simulink model "lugre_stick_slip"  (R2023a)
settings: Solver=FixedStepAuto  StartTime=0.0  StopTime=50  FixedStep=1e-4  RelTol=1e-3
values from neighbouring files (symbols this model uses):
  Ac = [0 1; 0 0]    [LuGre_parameters.m]
  alpha = 1    [LuGre_parameters.m]
  Fc = 2.94    [LuGre_parameters.m]
  Fs = 5.88    [LuGre_parameters.m]
  k = 2    [LuGre_parameters.m]
  Kstfb = [place(Ac,Bc,[-35,-30]),0]    [LuGre_parameters.m]
  m = 1    [LuGre_parameters.m]
  sigma0 = 2900    [LuGre_parameters.m]
  sigma1 = 107    [LuGre_parameters.m]
  sigma2 = 0    [LuGre_parameters.m]
  vs = 0.1    [LuGre_parameters.m]
libraries: slpidlib x1, simulink x1
settings Model: Creator=Alex  LastModifiedBy=Alex

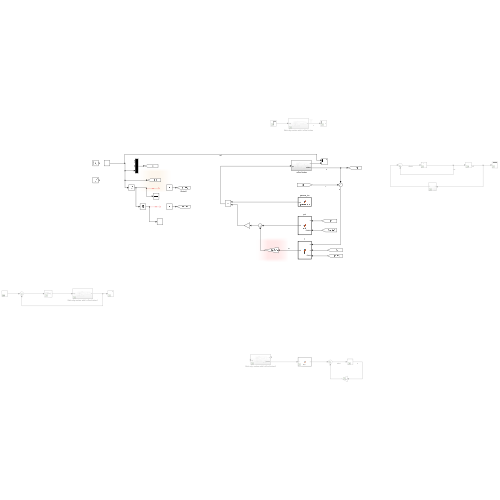
[thumbnail: Simulink's stored preview of the top-level diagram]
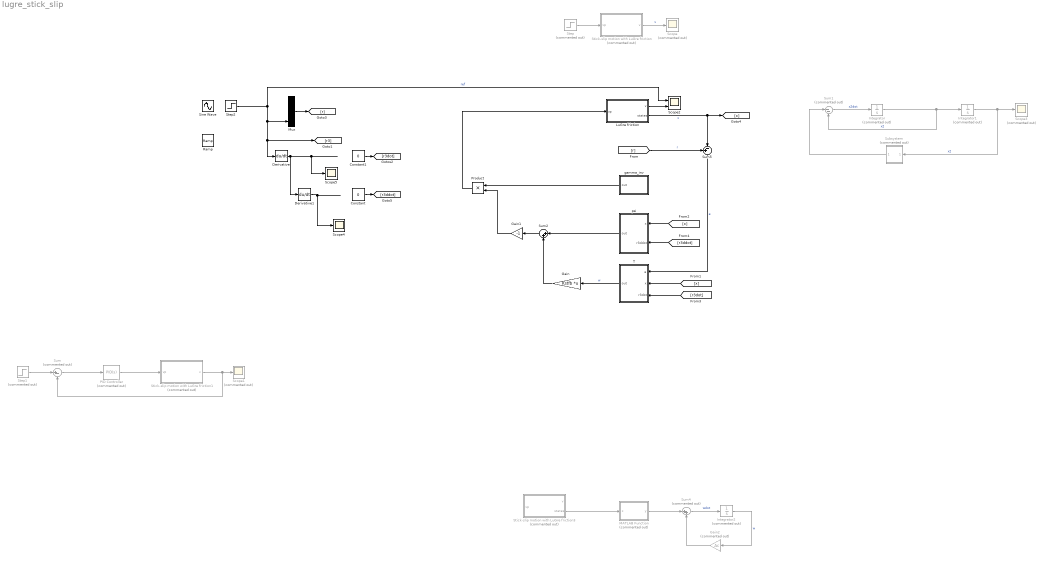
== system lugre_stick_slip ==
  Constant : Constant  Value=0
  Constant1 : Constant  Value=0
  Derivative : Derivative
  Derivative1 : Derivative
  Gain : Gain  Gain=Kstfb  Multiplication=Matrix(K*u)
  Gain1 : Gain  Gain=-1
  Gain2 : Gain  Commented=on  Gain=Ac
  Integrator : Integrator  Commented=on
  Integrator1 : Integrator  Commented=on
  Integrator2 : Integrator  Commented=on
  LuGre friction : Subsystem
  MATLAB Function : MATLAB Function  Commented=on  TreatAsAtomicUnit=on
  Mux : Mux  Inputs=3
  PID Controller : slpidlib/PID Controller  Commented=on  Controller=PID  Form=Parallel  TimeDomain=Continuous-time  UseExternalTs=off  SampleTime=-1  IntegratorMethod=Forward Euler  FilterMethod=Forward Euler  ControllerParametersSource=internal  P=4497.03009400386  I=153484.021687278  UseKiTs=off  D=32.6792113666645  N=9061.11275145139  UseFilter=on  TunerSelectOption=Transfer Function Based (PID Tuner App)  InitialConditionSource=internal  InitialConditionForIntegrator=0  InitialConditionForFilter=0  DifferentiatorICPrevScaledInput=0  ExternalReset=none  TrackingMode=off  Kt=1  LimitOutput=off  SatLimitsSource=internal  UpperSaturationLimit=inf  LowerSaturationLimit=-inf  LinearizeAsGain=on  AntiWindupMode=none  Kb=1  LimitIntegrator=off  UpperIntegratorSaturationLimit=inf  LowerIntegratorSaturationLimit=-inf  POutMin=[]  POutMax=[]  IOutMin=[]  IOutMax=[]  DOutMin=[]  DOutMax=[]  NOutMin=[]  NOutMax=[]  SumOutMin=[]  SumOutMax=[]  SaturationOutMin=[]  SaturationOutMax=[]  PParamMin=[]  PParamMax=[]  IParamMin=[]  IParamMax=[]  DParamMin=[]  DParamMax=[]  NParamMin=[]  NParamMax=[]  KbParamMin=[]  KbParamMax=[]  KtParamMin=[]  KtParamMax=[]  KbOutMin=[]  KbOutMax=[]  KtOutMin=[]  KtOutMax=[]  IntegratorOutMin=[]  IntegratorOutMax=[]  FilterOutMin=[]  FilterOutMax=[]  SumI1OutMin=[]  SumI1OutMax=[]  SumI2OutMin=[]  SumI2OutMax=[]  SumI3OutMin=[]  SumI3OutMax=[]  SumI4OutMin=[]  SumI4OutMax=[]  SumDOutMin=[]  SumDOutMax=[]  DifferentiatorOutMin=[]  DifferentiatorOutMax=[]  FilterDiffOutCoefMin=[]  FilterDiffOutCoefMax=[]  ReciprocalOutMin=[]  ReciprocalOutMax=[]  SumDenOutMin=[]  SumDenOutMax=[]  SumNumOutMin=[]  SumNumOutMax=[]  DivideOutMin=[]  DivideOutMax=[]  UdiffTsProdOutMin=[]  UdiffTsProdOutMax=[]  NTsProdOutMin=[]  NTsProdOutMax=[]  UintegralTsProdOutMin=[]  UintegralTsProdOutMax=[]  UngainTsProdOutMin=[]  UngainTsProdOutMax=[]  ClampingZeroOutDataTypeStr=Inherit: Inherit via back propagation  ClampingZeroOutMin=[]  ClampingZeroOutMax=[]  FilterDenConstantOutDataTypeStr=Inherit: Inherit via back propagation  FilterDenConstantOutMin=[]  FilterDenConstantOutMax=[]  PCopyOutDataTypeStr=Inherit: Inherit via back propagation  PCopyOutMin=[]  PCopyOutMax=[]  NCopyOutDataTypeStr=Inherit: Inherit via back propagation  NCopyOutMin=[]  NCopyOutMax=[]  IntegratorContinuousStateAttributes=''  IntegratorStateMustResolveToSignalObject=off  IntegratorRTWStateStorageClass=Auto  FilterContinuousStateAttributes=''  FilterStateMustResolveToSignalObject=off  FilterRTWStateStorageClass=Auto  ParallelPVariant=InternalParameters  IdealPVariant=Disabled  IVariant=InternalParameters  DVariant=InternalParameters  IntegratorVariant=Continuous  SatVariant=Disabled  AWVariant=Passthrough  PCopyVariant=Disabled  TRVariant=Disabled  FdbkBlocksVariant=Forward  IdealPFdbkVariant=Disabled  SatFdbkVariant=Disabled  DerivativeFilterVariant=ContFilter  NVariant=InternalParameters  NCopyVariant=Disabled  FilterICVariant=InternalICsFilter  IntegratorICVariant=InternalICs  ExternalResetVariant=Disabled  TRSumVariant=Passthrough  SumFdbkVariant=Disabled  SumVariant=Sum_PID  TsampFilterVariant=InternalTs  TsampNgainVariant=Passthrough  TsampIntegralVariant=Disabled_SignalSpec  ExternalSaturationOutDataTypeStr=Inherit: Same as second input
  Product : Product
  Ramp : simulink/Sources/Ramp  slope=1e-3  start=0  InitialOutput=0
  Scope : Scope  Commented=on
  Scope1 : Scope  Commented=on
  Scope2 : Scope  NumInputPorts=2
  Scope3 : Scope  Commented=on
  Scope4 : Scope
  Scope5 : Scope
  Sine Wave : Sin  Frequency=0.1  SampleTime=0
  Step : Step  Commented=on  Time=0  After=2  SampleTime=0
  Step1 : Step  Commented=on  Time=5  Before=2  After=3  SampleTime=0
  Step2 : Step  Time=0  After=10  SampleTime=0
  Stick-slip motion with LuGre friction : Subsystem  Commented=on
  Stick-slip motion with LuGre friction1 : Subsystem  Commented=on
  Stick-slip motion with LuGre friction3 : Subsystem  Commented=on
  Subsystem : Subsystem  Commented=on
  Sum : Sum  Commented=on  Inputs=|+-
  Sum1 : Sum  Commented=on  Inputs=|--
  Sum2 : Sum  Inputs=|++
  Sum4 : Sum  Commented=on  Inputs=|++
  Sum5 : Sum  Inputs=+-|
  T : MATLAB Function  TreatAsAtomicUnit=on
  gamma_inv : MATLAB Function  TreatAsAtomicUnit=on
  psi : MATLAB Function  TreatAsAtomicUnit=on
  wires:
  Step/1 -> Stick-slip motion with LuGre friction/1(vp)
  Stick-slip motion with LuGre friction/1(v) -> Scope/1  "v"
  Stick-slip motion with LuGre friction1/1(v) -> Sum/2, Scope1/1
  Sum/1 -> PID Controller/1
  PID Controller/1 -> Stick-slip motion with LuGre friction1/1(vp)
  Step1/1 -> Sum/1
  LuGre friction/1(v) -> Scope2/2
  Integrator/1 -> Integrator1/1, Sum1/2  "x2"
  Sum1/1 -> Integrator/1  "x2dot"
  Integrator1/1 -> Subsystem/1(In1), Scope3/1  "x2"
  Subsystem/1(Out1) -> Sum1/1
  Sum5/1 -> T/1(e)  "e"
  T/1(out) -> Gain/1  "w"
  psi/1(out) -> Sum2/1
  Gain/1 -> Sum2/2
  Sum2/1 -> Gain1/1
  gamma_inv/1(out) -> Product/1
  Gain1/1 -> Product/2
  Product/1 -> LuGre friction/1(vp)
  Sum4/1 -> Integrator2/1  "wdot"
  Integrator2/1 -> Gain2/1  "w"
  Gain2/1 -> Sum4/2
  MATLAB Function/1(y) -> Sum4/1
  Stick-slip motion with LuGre friction3/2(states) -> MATLAB Function/1(x)
  Step2/1 -> Scope2/1, [r3], Derivative/1, Mux/3  "ref"
  Mux/1 -> [r]
  [r] -> Sum5/1  "r"
  LuGre friction/2(states) -> Sum5/2, [x]  "x"
  [x] -> T/2(x)
  [x] -> psi/1(x)
  Derivative/1 -> Scope5/1, Derivative1/1
  Derivative1/1 -> Scope4/1
  [r3dot] -> T/3(r3dot)
  [r3ddot] -> psi/2(r3ddot)
  Constant/1 -> [r3ddot]
  Constant1/1 -> [r3dot]

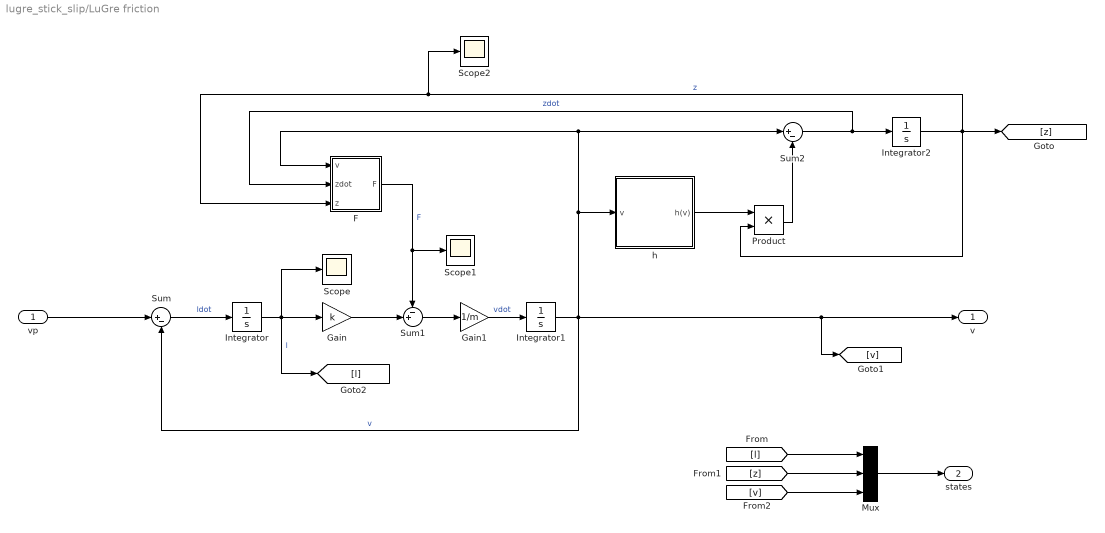
== system lugre_stick_slip/LuGre friction ==
  vp : Inport
  F : Subsystem
  Gain : Gain  Gain=k
  Gain1 : Gain  Gain=1/m
  Integrator : Integrator
  Integrator1 : Integrator
  Integrator2 : Integrator
  Mux : Mux  Inputs=3
  Product : Product
  Scope : Scope
  Scope1 : Scope
  Scope2 : Scope
  Sum : Sum  Inputs=|+-
  Sum1 : Sum  Inputs=-+|
  Sum2 : Sum  Inputs=|+-
  h : Subsystem
  v : Outport
  states : Outport  Port=2
  wires:
  Product/1 -> Sum2/2
  h/1(h(v)) -> Product/1
  Integrator2/1 -> F/3(z), Scope2/1, [z], Product/2  "z"
  F/1(F) -> Scope1/1, Sum1/1  "F"
  Sum2/1 -> Integrator2/1, F/2(zdot)  "zdot"
  vp/1 -> Sum/1
  Sum1/1 -> Gain1/1
  Sum/1 -> Integrator/1  "ldot"
  Integrator1/1 -> [v], v/1, h/1(v), Sum2/1, F/1(v), Sum/2  "v"
  Gain1/1 -> Integrator1/1  "vdot"
  Gain/1 -> Sum1/2
  Integrator/1 -> [l], Gain/1, Scope/1  "l"
  Mux/1 -> states/1
  [l] -> Mux/1
  [v] -> Mux/3
  [z] -> Mux/2

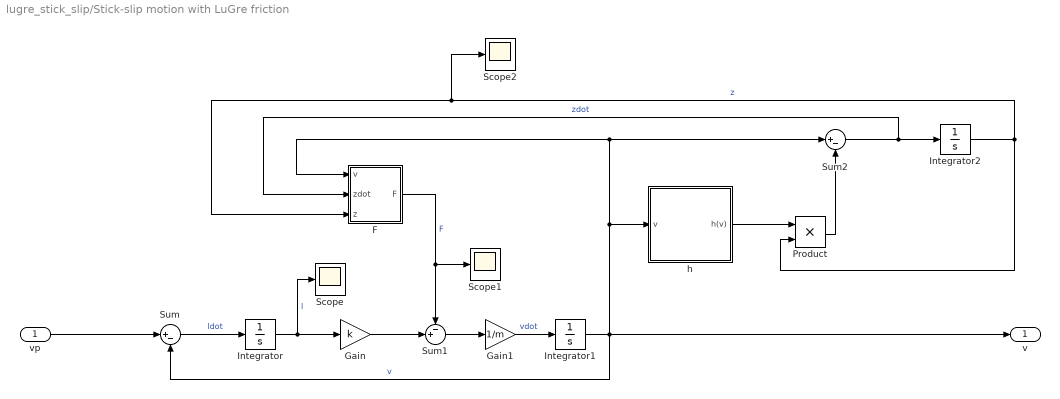
== system lugre_stick_slip/Stick-slip motion with LuGre friction ==
  vp : Inport
  F : Subsystem
  Gain : Gain  Gain=k
  Gain1 : Gain  Gain=1/m
  Integrator : Integrator
  Integrator1 : Integrator
  Integrator2 : Integrator
  Product : Product
  Scope : Scope
  Scope1 : Scope
  Scope2 : Scope
  Sum : Sum  Inputs=|+-
  Sum1 : Sum  Inputs=-+|
  Sum2 : Sum  Inputs=|+-
  h : Subsystem
  v : Outport
  wires:
  Integrator/1 -> Scope/1, Gain/1  "l"
  Gain/1 -> Sum1/2
  Gain1/1 -> Integrator1/1  "vdot"
  Integrator1/1 -> Sum/2, F/1(v), Sum2/1, h/1(v), v/1  "v"
  Sum/1 -> Integrator/1  "ldot"
  Sum1/1 -> Gain1/1
  vp/1 -> Sum/1
  Sum2/1 -> F/2(zdot), Integrator2/1  "zdot"
  F/1(F) -> Sum1/1, Scope1/1  "F"
  Integrator2/1 -> Product/2, Scope2/1, F/3(z)  "z"
  h/1(h(v)) -> Product/1
  Product/1 -> Sum2/2

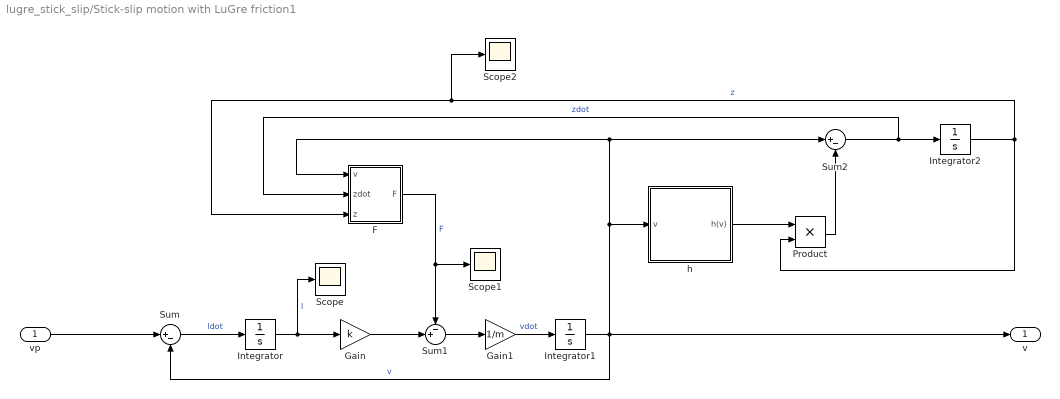
== system lugre_stick_slip/Stick-slip motion with LuGre friction1 ==
  vp : Inport
  F : Subsystem
  Gain : Gain  Gain=k
  Gain1 : Gain  Gain=1/m
  Integrator : Integrator
  Integrator1 : Integrator
  Integrator2 : Integrator
  Product : Product
  Scope : Scope
  Scope1 : Scope
  Scope2 : Scope
  Sum : Sum  Inputs=|+-
  Sum1 : Sum  Inputs=-+|
  Sum2 : Sum  Inputs=|+-
  h : Subsystem
  v : Outport
  wires:
  Product/1 -> Sum2/2
  h/1(h(v)) -> Product/1
  Integrator2/1 -> F/3(z), Scope2/1, Product/2  "z"
  F/1(F) -> Scope1/1, Sum1/1  "F"
  Sum2/1 -> Integrator2/1, F/2(zdot)  "zdot"
  vp/1 -> Sum/1
  Sum1/1 -> Gain1/1
  Sum/1 -> Integrator/1  "ldot"
  Integrator1/1 -> v/1, h/1(v), Sum2/1, F/1(v), Sum/2  "v"
  Gain1/1 -> Integrator1/1  "vdot"
  Gain/1 -> Sum1/2
  Integrator/1 -> Gain/1, Scope/1  "l"

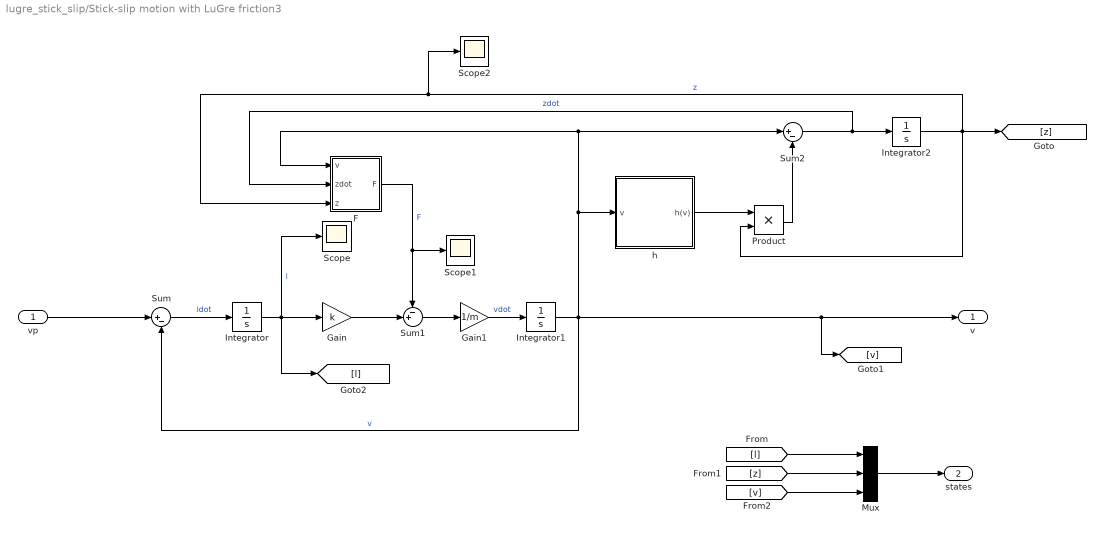
== system lugre_stick_slip/Stick-slip motion with LuGre friction3 ==
  vp : Inport
  F : Subsystem
  Gain : Gain  Gain=k
  Gain1 : Gain  Gain=1/m
  Integrator : Integrator  InitialCondition=3
  Integrator1 : Integrator  InitialCondition=7
  Integrator2 : Integrator
  Mux : Mux  Inputs=3
  Product : Product
  Scope : Scope
  Scope1 : Scope
  Scope2 : Scope
  Sum : Sum  Inputs=|+-
  Sum1 : Sum  Inputs=-+|
  Sum2 : Sum  Inputs=|+-
  h : Subsystem
  v : Outport
  states : Outport  Port=2
  wires:
  [z] -> Mux/2
  [v] -> Mux/3
  [l] -> Mux/1
  Mux/1 -> states/1
  Integrator/1 -> Scope/1, Gain/1, [l]  "l"
  Gain/1 -> Sum1/2
  Gain1/1 -> Integrator1/1  "vdot"
  Integrator1/1 -> Sum/2, F/1(v), Sum2/1, h/1(v), v/1, [v]  "v"
  Sum/1 -> Integrator/1  "ldot"
  Sum1/1 -> Gain1/1
  vp/1 -> Sum/1
  Sum2/1 -> F/2(zdot), Integrator2/1  "zdot"
  F/1(F) -> Sum1/1, Scope1/1  "F"
  Integrator2/1 -> Product/2, [z], Scope2/1, F/3(z)  "z"
  h/1(h(v)) -> Product/1
  Product/1 -> Sum2/2

== system lugre_stick_slip/Subsystem ==
  In1 : Inport
  Out1 : Outport
  wires:
  In1/1 -> Out1/1

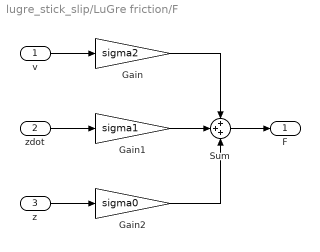
== system lugre_stick_slip/LuGre friction/F ==
  v : Inport
  zdot : Inport  Port=2
  z : Inport  Port=3
  Gain : Gain  Gain=sigma2
  Gain1 : Gain  Gain=sigma1
  Gain2 : Gain  Gain=sigma0
  Sum : Sum  Inputs=+++
  F : Outport
  wires:
  Gain2/1 -> Sum/3
  Gain1/1 -> Sum/2
  z/1 -> Gain2/1
  zdot/1 -> Gain1/1
  Gain/1 -> Sum/1
  Sum/1 -> F/1
  v/1 -> Gain/1

== system lugre_stick_slip/LuGre friction/h ==
  v : Inport
  Abs : Abs  SaturateOnIntegerOverflow=off
  Divide : Product  Inputs=*/
  Gain : Gain  Gain=sigma0
  g : Subsystem
  h(v) : Outport
  wires:
  Gain/1 -> h(v)/1
  Divide/1 -> Gain/1
  g/1(g(v)) -> Divide/2
  Abs/1 -> Divide/1
  v/1 -> Abs/1, g/1(v)

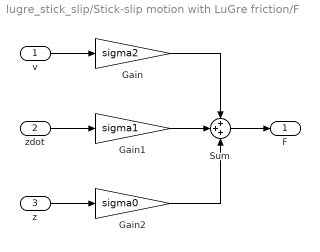
== system lugre_stick_slip/Stick-slip motion with LuGre friction/F ==
  v : Inport
  zdot : Inport  Port=2
  z : Inport  Port=3
  Gain : Gain  Gain=sigma2
  Gain1 : Gain  Gain=sigma1
  Gain2 : Gain  Gain=sigma0
  Sum : Sum  Inputs=+++
  F : Outport
  wires:
  v/1 -> Gain/1
  Sum/1 -> F/1
  Gain/1 -> Sum/1
  zdot/1 -> Gain1/1
  z/1 -> Gain2/1
  Gain1/1 -> Sum/2
  Gain2/1 -> Sum/3

== system lugre_stick_slip/Stick-slip motion with LuGre friction/h ==
  v : Inport
  Abs : Abs  SaturateOnIntegerOverflow=off
  Divide : Product  Inputs=*/
  Gain : Gain  Gain=sigma0
  g : Subsystem
  h(v) : Outport
  wires:
  v/1 -> g/1(v), Abs/1
  Abs/1 -> Divide/1
  g/1(g(v)) -> Divide/2
  Divide/1 -> Gain/1
  Gain/1 -> h(v)/1

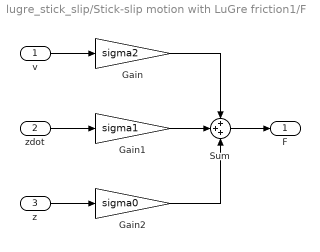
== system lugre_stick_slip/Stick-slip motion with LuGre friction1/F ==
  v : Inport
  zdot : Inport  Port=2
  z : Inport  Port=3
  Gain : Gain  Gain=sigma2
  Gain1 : Gain  Gain=sigma1
  Gain2 : Gain  Gain=sigma0
  Sum : Sum  Inputs=+++
  F : Outport
  wires:
  Gain2/1 -> Sum/3
  Gain1/1 -> Sum/2
  z/1 -> Gain2/1
  zdot/1 -> Gain1/1
  Gain/1 -> Sum/1
  Sum/1 -> F/1
  v/1 -> Gain/1

== system lugre_stick_slip/Stick-slip motion with LuGre friction1/h ==
  v : Inport
  Abs : Abs  SaturateOnIntegerOverflow=off
  Divide : Product  Inputs=*/
  Gain : Gain  Gain=sigma0
  g : Subsystem
  h(v) : Outport
  wires:
  Gain/1 -> h(v)/1
  Divide/1 -> Gain/1
  g/1(g(v)) -> Divide/2
  Abs/1 -> Divide/1
  v/1 -> Abs/1, g/1(v)

== system lugre_stick_slip/Stick-slip motion with LuGre friction3/F ==
  v : Inport
  zdot : Inport  Port=2
  z : Inport  Port=3
  Gain : Gain  Gain=sigma2
  Gain1 : Gain  Gain=sigma1
  Gain2 : Gain  Gain=sigma0
  Sum : Sum  Inputs=+++
  F : Outport
  wires:
  v/1 -> Gain/1
  Sum/1 -> F/1
  Gain/1 -> Sum/1
  zdot/1 -> Gain1/1
  z/1 -> Gain2/1
  Gain1/1 -> Sum/2
  Gain2/1 -> Sum/3

== system lugre_stick_slip/Stick-slip motion with LuGre friction3/h ==
  v : Inport
  Abs : Abs  SaturateOnIntegerOverflow=off
  Divide : Product  Inputs=*/
  Gain : Gain  Gain=sigma0
  g : Subsystem
  h(v) : Outport
  wires:
  v/1 -> g/1(v), Abs/1
  Abs/1 -> Divide/1
  g/1(g(v)) -> Divide/2
  Divide/1 -> Gain/1
  Gain/1 -> h(v)/1

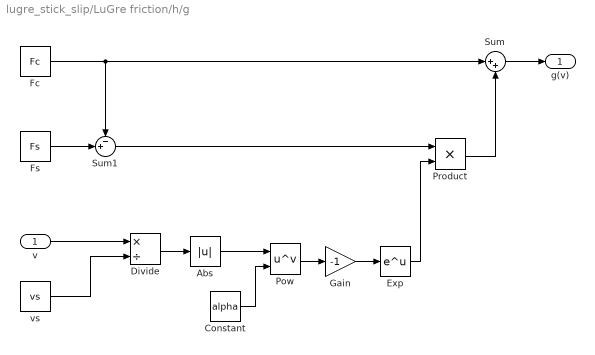
== system lugre_stick_slip/LuGre friction/h/g ==
  v : Inport
  Abs : Abs  SaturateOnIntegerOverflow=off
  Constant : Constant  Value=alpha
  Divide : Product  Inputs=*/
  Exp : Math
  Fc : Constant  Value=Fc
  Fs : Constant  Value=Fs
  Gain : Gain  Gain=-1
  Pow : Math  Operator=pow  RndMeth=Zero
  Product : Product
  Sum : Sum  Inputs=|++
  Sum1 : Sum  Inputs=-+|
  vs : Constant  Value=vs
  g(v) : Outport
  wires:
  Sum/1 -> g(v)/1
  Product/1 -> Sum/2
  Exp/1 -> Product/2
  Gain/1 -> Exp/1
  Pow/1 -> Gain/1
  Constant/1 -> Pow/2
  Abs/1 -> Pow/1
  Divide/1 -> Abs/1
  vs/1 -> Divide/2
  v/1 -> Divide/1
  Sum1/1 -> Product/1
  Fs/1 -> Sum1/2
  Fc/1 -> Sum/1, Sum1/1

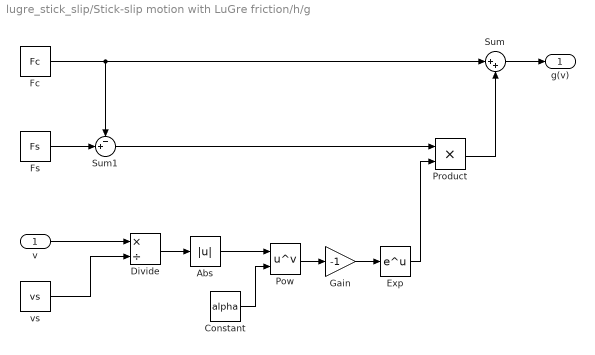
== system lugre_stick_slip/Stick-slip motion with LuGre friction/h/g ==
  v : Inport
  Abs : Abs  SaturateOnIntegerOverflow=off
  Constant : Constant  Value=alpha
  Divide : Product  Inputs=*/
  Exp : Math
  Fc : Constant  Value=Fc
  Fs : Constant  Value=Fs
  Gain : Gain  Gain=-1
  Pow : Math  Operator=pow  RndMeth=Zero
  Product : Product
  Sum : Sum  Inputs=|++
  Sum1 : Sum  Inputs=-+|
  vs : Constant  Value=vs
  g(v) : Outport
  wires:
  Fc/1 -> Sum1/1, Sum/1
  Fs/1 -> Sum1/2
  Sum1/1 -> Product/1
  v/1 -> Divide/1
  vs/1 -> Divide/2
  Divide/1 -> Abs/1
  Abs/1 -> Pow/1
  Constant/1 -> Pow/2
  Pow/1 -> Gain/1
  Gain/1 -> Exp/1
  Exp/1 -> Product/2
  Product/1 -> Sum/2
  Sum/1 -> g(v)/1

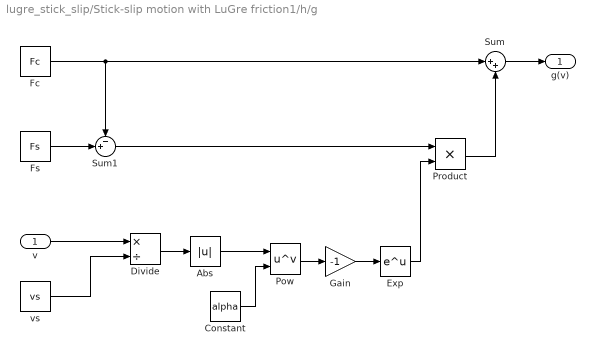
== system lugre_stick_slip/Stick-slip motion with LuGre friction1/h/g ==
  v : Inport
  Abs : Abs  SaturateOnIntegerOverflow=off
  Constant : Constant  Value=alpha
  Divide : Product  Inputs=*/
  Exp : Math
  Fc : Constant  Value=Fc
  Fs : Constant  Value=Fs
  Gain : Gain  Gain=-1
  Pow : Math  Operator=pow  RndMeth=Zero
  Product : Product
  Sum : Sum  Inputs=|++
  Sum1 : Sum  Inputs=-+|
  vs : Constant  Value=vs
  g(v) : Outport
  wires:
  Sum/1 -> g(v)/1
  Product/1 -> Sum/2
  Exp/1 -> Product/2
  Gain/1 -> Exp/1
  Pow/1 -> Gain/1
  Constant/1 -> Pow/2
  Abs/1 -> Pow/1
  Divide/1 -> Abs/1
  vs/1 -> Divide/2
  v/1 -> Divide/1
  Sum1/1 -> Product/1
  Fs/1 -> Sum1/2
  Fc/1 -> Sum/1, Sum1/1

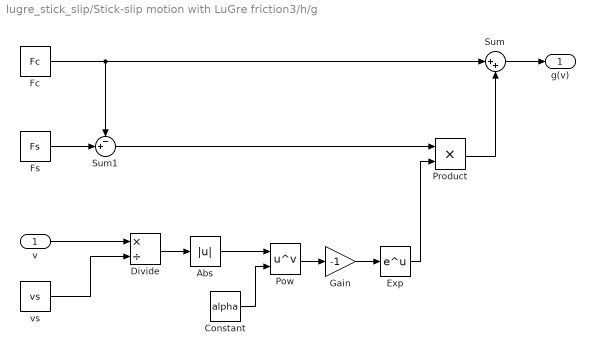
== system lugre_stick_slip/Stick-slip motion with LuGre friction3/h/g ==
  v : Inport
  Abs : Abs  SaturateOnIntegerOverflow=off
  Constant : Constant  Value=alpha
  Divide : Product  Inputs=*/
  Exp : Math
  Fc : Constant  Value=Fc
  Fs : Constant  Value=Fs
  Gain : Gain  Gain=-1
  Pow : Math  Operator=pow  RndMeth=Zero
  Product : Product
  Sum : Sum  Inputs=|++
  Sum1 : Sum  Inputs=-+|
  vs : Constant  Value=vs
  g(v) : Outport
  wires:
  Fc/1 -> Sum1/1, Sum/1
  Fs/1 -> Sum1/2
  Sum1/1 -> Product/1
  v/1 -> Divide/1
  vs/1 -> Divide/2
  Divide/1 -> Abs/1
  Abs/1 -> Pow/1
  Constant/1 -> Pow/2
  Pow/1 -> Gain/1
  Gain/1 -> Exp/1
  Exp/1 -> Product/2
  Product/1 -> Sum/2
  Sum/1 -> g(v)/1

== matlab function lugre_stick_slip/T ==
  data: e input; out output; x input; r3dot input
function out = T(e, x, r3dot)
    arguments
        e (3,1) {mustBeNumeric}
        x (3,1) {mustBeNumeric}
        r3dot
    end
m=1;
k=2;
alpha=1;
sigma0=2900;%3.9e4;
sigma1=107;%395;
sigma2=0;
Fc=2.94;
Fs=5.88;
vs=0.1;%0.01;v

A=abs(e(3))/(Fc+(Fs-Fc)*exp(-(abs(x(3)/vs))^alpha));
out =[m*e(3);...
    e(3);...
    r3dot-1/m*(k*x(1)-(sigma1+sigma2)*x(3)-sigma0*x(2).*(1-sigma1*A))];

== matlab function lugre_stick_slip/gamma_inv ==
  data: out output
function out = gamma_inv()
m=1;
k=2;
alpha=1;
sigma0=2900;%3.9e4;
sigma1=107;%395;
sigma2=0;
Fc=2.94;
Fs=5.88;
vs=0.1;%0.01;

out = -m/k;

== matlab function lugre_stick_slip/MATLAB Function ==
  data: x input; y output
function y = fcn(x)

y = u;

== matlab function lugre_stick_slip/psi ==
  data: out output; x input; r3ddot input
function out = psi(x, r3ddot)

    arguments
        x (3,1) {mustBeNumeric}
        r3ddot
    end

m=1;
k=2;
alpha=1;
sigma0=2900;%3.9e4;
sigma1=107;%395;
sigma2=0;
Fc=2.94;
Fs=5.88;
vs=0.1;%0.01;

x3=x(3);
A=abs(x3)/(Fc+(Fs-Fc)*exp(-(abs(x3/vs))^alpha));
x3dot=1/m*(k*x(1)-(sigma1+sigma2)*x3-sigma0*x(2).*(1-sigma1*A));
out = r3ddot+(sigma1+sigma2)/m*x3dot...
    +(k+sigma0)/m*x3...
    -sigma0*sigma1/m*x3.*A...
    -sigma0^2/m*x(2).*A...
    +sigma0^2*sigma1/m*x(2).*A.*A...
    -sigma0*sigma1/m*x(2).*x3dot...
    .*(sign(x3).*(1+alpha/(vs)^alpha*(abs(x3))^alpha)/(Fc+(Fs-Fc)*exp(-(abs(x3/vs))^alpha)));
